simulink model "tire_parameter_estimation"  (R2024b)
settings: Solver=VariableStepAuto  StartTime=0.0  StopTime=time(end)  MaxStep=1/60  RelTol=1e-3
InitFcn:
  | tire_parameter_estimation_init;
values from neighbouring files (symbols this model uses):
  IC = sf.*x_mes{k}(1,:)    [lateral_ui_validation.m]    (also in lateral_validation.m; lateral_validation_lpv.m; longitudinal_validation.m; longitudinal_validation_lpv.m)
  kfyaf = params(12)    [tire_parameter_estimation_init.m]
  kfyar = params(13)    [tire_parameter_estimation_init.m]
  kfylf = params(14)    [tire_parameter_estimation_init.m]
  kfylr = params(15)    [tire_parameter_estimation_init.m]
  kmzaf = 0.65798    [tire_parameter_estimation_init.m]
  kmzar = 5.6439    [tire_parameter_estimation_init.m]
  kmzlf = 0.03128    [tire_parameter_estimation_init.m]
  kmzlr = 0.97436    [tire_parameter_estimation_init.m]
  params = @(v)s2m(bikeSimToPrydeParameters(bs,v/3.6))    [lateral_linear_analysis.m]    (also in lateral_ui_validation.m; lateral_validation.m; lateral_validation_lpv.m; longitudinal_linear_analysis.m)
libraries: simulink_extras x2
settings Model: Creator=marti  LastModifiedBy=marti

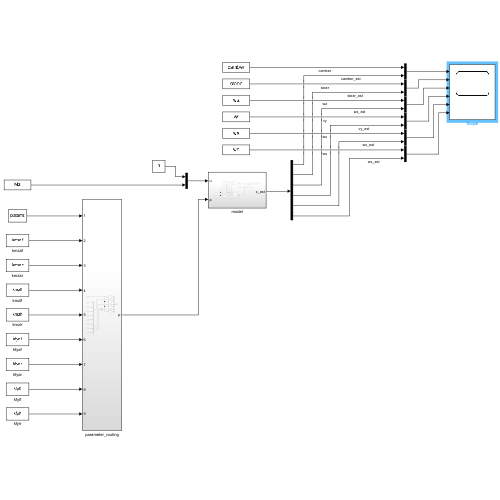
[thumbnail: Simulink's stored preview of the top-level diagram]
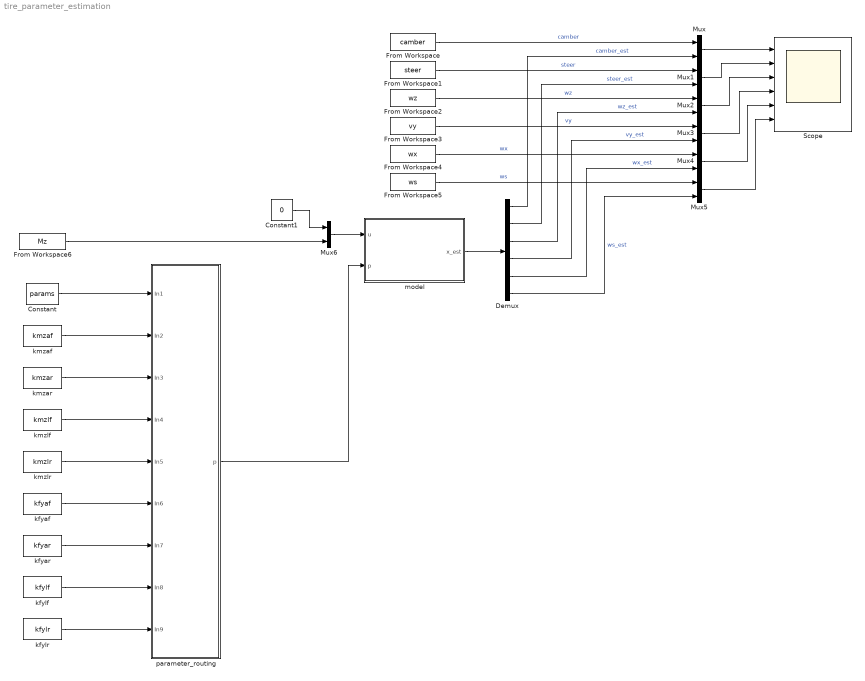
== system tire_parameter_estimation ==
  Constant : Constant  Value=params
  Constant1 : Constant  Value=0
  Demux : Demux  Outputs=6
  From Workspace : FromWorkspace  VariableName=camber
  From Workspace1 : FromWorkspace  VariableName=steer
  From Workspace2 : FromWorkspace  VariableName=wz
  From Workspace3 : FromWorkspace  VariableName=vy
  From Workspace4 : FromWorkspace  VariableName=wx
  From Workspace5 : FromWorkspace  VariableName=ws
  From Workspace6 : FromWorkspace  VariableName=Mz
  Mux{,1..6} (7 alike) : Mux  Inputs=2
  Scope : Scope  NumInputPorts=6
  kfyaf : Constant  Value=kfyaf
  kfyar : Constant  Value=kfyar
  kfylf : Constant  Value=kfylf
  kfylr : Constant  Value=kfylr
  kmzaf : Constant  Value=kmzaf
  kmzar : Constant  Value=kmzar
  kmzlf : Constant  Value=kmzlf
  kmzlr : Constant  Value=kmzlr
  model : Subsystem
  parameter_routing : Subsystem
  wires:
  Constant/1 -> parameter_routing/1(In1)
  kmzaf/1 -> parameter_routing/2(In2)
  kmzar/1 -> parameter_routing/3(In3)
  kmzlf/1 -> parameter_routing/4(In4)
  kmzlr/1 -> parameter_routing/5(In5)
  kfyaf/1 -> parameter_routing/6(In6)
  kfyar/1 -> parameter_routing/7(In7)
  kfylf/1 -> parameter_routing/8(In8)
  kfylr/1 -> parameter_routing/9(In9)
  parameter_routing/1(p) -> model/2(p)
  model/1(x_est) -> Demux/1
  Mux/1 -> Scope/1
  Mux1/1 -> Scope/2
  Mux2/1 -> Scope/3
  Mux3/1 -> Scope/4
  Mux5/1 -> Scope/6
  Mux4/1 -> Scope/5
  From Workspace/1 -> Mux/1  "camber"
  From Workspace1/1 -> Mux1/1  "steer"
  From Workspace2/1 -> Mux2/1  "wz"
  From Workspace3/1 -> Mux3/1  "vy"
  From Workspace4/1 -> Mux4/1  "wx"
  From Workspace5/1 -> Mux5/1  "ws"
  Demux/1 -> Mux/2  "camber_est"
  Demux/2 -> Mux1/2  "steer_est"
  Demux/3 -> Mux2/2  "wz_est"
  Demux/4 -> Mux3/2  "vy_est"
  Demux/5 -> Mux4/2  "wx_est"
  Demux/6 -> Mux5/2  "ws_est"
  Mux6/1 -> model/1(u)
  From Workspace6/1 -> Mux6/2
  Constant1/1 -> Mux6/1

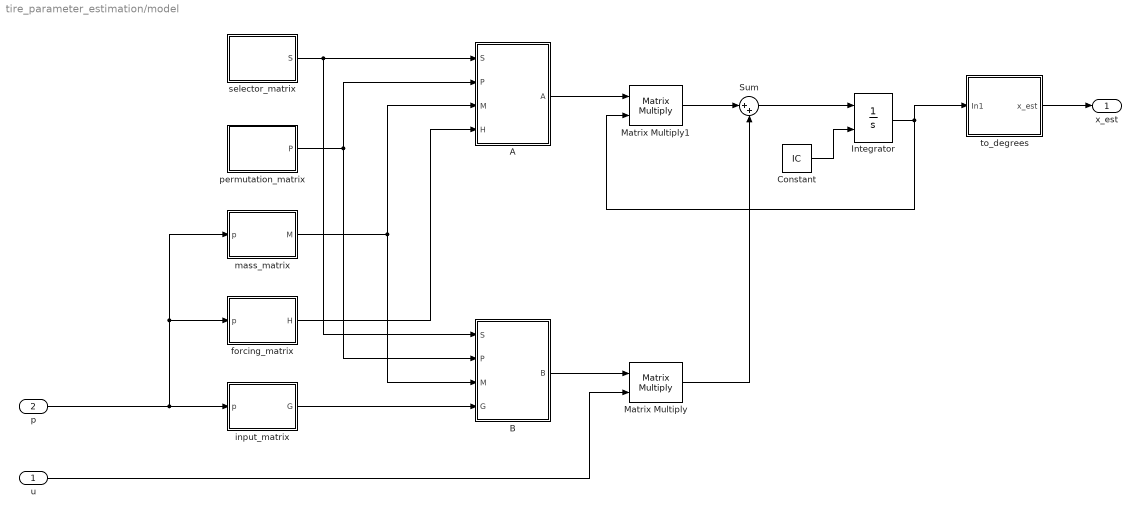
== system tire_parameter_estimation/model ==
  u : Inport
  p : Inport  Port=2
  A : MATLAB Function  TreatAsAtomicUnit=on
  B : MATLAB Function  TreatAsAtomicUnit=on
  Constant : Constant  Value=IC
  Integrator : Integrator  InitialConditionSource=external
  Matrix Multiply : Product  Multiplication=Matrix(*)
  Matrix Multiply1 : Product  Multiplication=Matrix(*)
  Sum : Sum  Inputs=|++
  forcing_matrix : MATLAB Function  TreatAsAtomicUnit=on
  input_matrix : MATLAB Function  TreatAsAtomicUnit=on
  mass_matrix : MATLAB Function  TreatAsAtomicUnit=on
  permutation_matrix : MATLAB Function  TreatAsAtomicUnit=on
  selector_matrix : MATLAB Function  TreatAsAtomicUnit=on
  to_degrees : Subsystem
  x_est : Outport
  wires:
  p/1 -> mass_matrix/1(p), forcing_matrix/1(p), input_matrix/1(p)
  Matrix Multiply1/1 -> Sum/1
  B/1(B) -> Matrix Multiply/1
  A/1(A) -> Matrix Multiply1/1
  selector_matrix/1(S) -> B/1(S), A/1(S)
  input_matrix/1(G) -> B/4(G)
  forcing_matrix/1(H) -> A/4(H)
  permutation_matrix/1(P) -> B/2(P), A/2(P)
  mass_matrix/1(M) -> B/3(M), A/3(M)
  Matrix Multiply/1 -> Sum/2
  Sum/1 -> Integrator/1
  u/1 -> Matrix Multiply/2
  Integrator/1 -> to_degrees/1(In1), Matrix Multiply1/2
  to_degrees/1(x_est) -> x_est/1
  Constant/1 -> Integrator/2

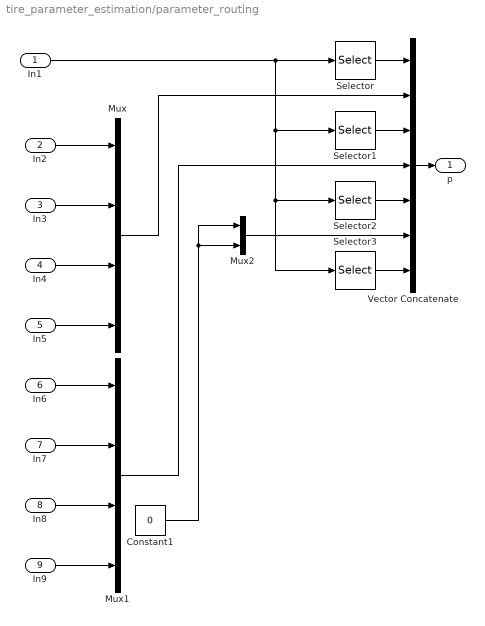
== system tire_parameter_estimation/parameter_routing ==
  In1 : Inport
  In2 : Inport  Port=2
  In3 : Inport  Port=3
  In4 : Inport  Port=4
  In5 : Inport  Port=5
  In6 : Inport  Port=6
  In7 : Inport  Port=7
  In8 : Inport  Port=8
  In9 : Inport  Port=9
  Constant1 : Constant  Value=0
  Mux : Mux
  Mux1 : Mux
  Mux2 : Mux  Inputs=2
  Selector : Selector  InputPortWidth=35  IndexOptions=Index vector (dialog)  Indices=1:6  OutputSizes=1
  Selector1 : Selector  InputPortWidth=35  IndexOptions=Index vector (dialog)  Indices=11  OutputSizes=1
  Selector2 : Selector  InputPortWidth=35  IndexOptions=Index vector (dialog)  Indices=16:26  OutputSizes=1
  Selector3 : Selector  InputPortWidth=35  IndexOptions=Index vector (dialog)  Indices=29:35  OutputSizes=1
  Vector Concatenate : Concatenate  NumInputs=7
  p : Outport
  wires:
  In8/1 -> Mux1/3
  Selector2/1 -> Vector Concatenate/5
  In1/1 -> Selector2/1, Selector3/1, Selector1/1, Selector/1
  In6/1 -> Mux1/1
  Selector3/1 -> Vector Concatenate/7
  Mux2/1 -> Vector Concatenate/6
  Selector/1 -> Vector Concatenate/1
  Constant1/1 -> Mux2/2, Mux2/1
  Selector1/1 -> Vector Concatenate/3
  In2/1 -> Mux/1
  Mux1/1 -> Vector Concatenate/4
  Mux/1 -> Vector Concatenate/2
  In7/1 -> Mux1/2
  Vector Concatenate/1 -> p/1
  In9/1 -> Mux1/4
  In5/1 -> Mux/4
  In4/1 -> Mux/3
  In3/1 -> Mux/2

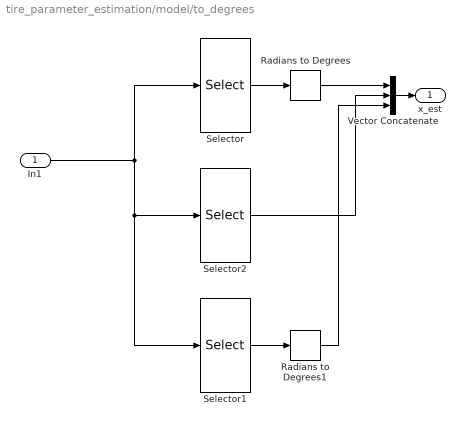
== system tire_parameter_estimation/model/to_degrees ==
  In1 : Inport
  Radians to Degrees : simulink_extras/Transformations/Radians to Degrees
  Radians to Degrees1 : simulink_extras/Transformations/Radians to Degrees
  Selector : Selector  InputPortWidth=6  IndexOptions=Index vector (dialog)  Indices=1:3  OutputSizes=1
  Selector1 : Selector  InputPortWidth=6  IndexOptions=Index vector (dialog)  Indices=5:6  OutputSizes=1
  Selector2 : Selector  InputPortWidth=6  IndexOptions=Index vector (dialog)  Indices=4  OutputSizes=1
  Vector Concatenate : Concatenate  NumInputs=3
  x_est : Outport
  wires:
  Selector1/1 -> Radians to Degrees1/1
  Selector2/1 -> Vector Concatenate/2
  Radians to Degrees/1 -> Vector Concatenate/1
  Selector/1 -> Radians to Degrees/1
  Radians to Degrees1/1 -> Vector Concatenate/3
  In1/1 -> Selector/1, Selector1/1, Selector2/1
  Vector Concatenate/1 -> x_est/1

== matlab function tire_parameter_estimation/model/permutation_matrix ==
  data: P output
function P = fcn()
P = prydeMotorcycleLateralPermutationMatrix();

== matlab function tire_parameter_estimation/model/selector_matrix ==
  data: S output
function S = fcn()
S = prydeMotorcycleLateralSelectorMatrix();

== matlab function tire_parameter_estimation/model/mass_matrix ==
  data: p input; M output
function M = fcn(p)
M = prydeMotorcycleLateralMassMatrix(p);

== matlab function tire_parameter_estimation/model/forcing_matrix ==
  data: p input; H output
function H = fcn(p)
H = prydeMotorcycleLateralForcingMatrix(p);

== matlab function tire_parameter_estimation/model/input_matrix ==
  data: p input; G output
function G = fcn(p)
G = prydeMotorcycleLateralInputMatrix(p);

== matlab function tire_parameter_estimation/model/A ==
  data: S input; P input; M input; A output; H input
function A = fcn(S,P,M,H)
A = S*P*(M\H)*S.';

== matlab function tire_parameter_estimation/model/B ==
  data: S input; P input; M input; B output; G input
function B = fcn(S,P,M,G)
B = S*P*(M\G);
